simulink model "EvilSpagetty"  (R2020b)
settings: Solver=VariableStepAuto  StartTime=0.0  StopTime=3  RelTol=1e-3
(part 5 of 7)

== matlab function EvilSpagetty/1//Mt ==
  data: u1 input; y output; u2 input; u3 input; u4 input; u5 input; u6 input; u7 input; u8 input; u9 input; u10 input
function y = fcn(u1,u2,u3,u4,u5,u6,u7,u8,u9,u10)
theta1=u6;
theta2=u7;
theta3=u8;
theta4=u9;
theta5=u10;
M=[(4725330594848641*cos(2*theta2))/288230376151711744 - (1393797*cos(2*theta3))/22300745198530623141535718272648361505980416 - (12544169*cos(2*theta4))/22300745198530623141535718272648361505980416 - (3240011242931075*cos(2*theta5))/73786976294838206464 + (3825825015716409*sin(2*theta2))/147573952589676412928 + (2282168433090971*sin(2*theta5))/37778931862957161709568 + (3257081095467945*cos(theta3))/288230376151711744 + (7220698343344529*cos(theta4))/2305843009213693952 - (7028085605816175*sin(theta3))/590295810358705651712 + (5387337053181017*cos(theta3)*cos(theta4))/1152921504606846976 + (5571380563941847*cos(theta5)*sin(theta4))/9223372036854775808 - (5387337053181017*sin(theta3)*sin(theta4))/1152921504606846976 - (7988070105025833*sin(theta4)*sin(theta5))/4722366482869645213696 + (3257081095467945*cos(2*theta2)*cos(theta3))/288230376151711744 - (13937967*cos(2*theta2)*cos(theta4))/2787593149816327892691964784081045188247552 - (13937967*cos(2*theta3)*cos(theta4))/2787593149816327892691964784081045188247552 - (7028085605816175*cos(2*theta2)*sin(theta3))/590295810358705651712 - (7028085605816175*sin(2*theta2)*cos(theta3))/590295810358705651712 + (2787593*sin(2*theta2)*cos(theta5))/5575186299632655785383929568162090376495104 + (2787593*sin(2*theta3)*cos(theta5))/5575186299632655785383929568162090376495104 + (2787593*sin(2*theta4)*cos(theta5))/5575186299632655785383929568162090376495104 - (3257081095467945*sin(2*theta2)*sin(theta3))/288230376151711744 + (13937965*sin(2*theta2)*sin(theta4))/2787593149816327892691964784081045188247552 - (2854495*sin(2*theta2)*sin(theta5))/5708990770823839524233143877797980545530986496 + (13937965*sin(2*theta3)*sin(theta4))/2787593149816327892691964784081045188247552 - (2854495*sin(2*theta3)*sin(theta5))/5708990770823839524233143877797980545530986496 - (2854495*sin(2*theta4)*sin(theta5))/5708990770823839524233143877797980545530986496 - (8356542075167085*cos(2*theta2)*cos(2*theta3))/2305843009213693952 - (11150375*cos(2*theta2)*cos(2*theta4))/178405961588244985132285746181186892047843328 - (1393797*cos(2*theta2)*cos(2*theta5))/22300745198530623141535718272648361505980416 - (11150375*cos(2*theta3)*cos(2*theta4))/178405961588244985132285746181186892047843328 - (1393797*cos(2*theta3)*cos(2*theta5))/22300745198530623141535718272648361505980416 - (1393797*cos(2*theta4)*cos(2*theta5))/22300745198530623141535718272648361505980416 - (1007824040173657*cos(2*theta2)*sin(2*theta3))/288230376151711744 - (1007824040173657*cos(2*theta3)*sin(2*theta2))/288230376151711744 - (17126969*cos(2*theta2)*sin(2*theta5))/91343852333181432387730302044767688728495783936 - (cos(2*theta5)*sin(2*theta2))/91343852333181432387730302044767688728495783936 - (17126969*cos(2*theta3)*sin(2*theta5))/91343852333181432387730302044767688728495783936 - (cos(2*theta5)*sin(2*theta3))/91343852333181432387730302044767688728495783936 - (17126969*cos(2*theta4)*sin(2*theta5))/91343852333181432387730302044767688728495783936 - (cos(2*theta5)*sin(2*theta4))/91343852333181432387730302044767688728495783936 + (8356542075167085*sin(2*theta2)*sin(2*theta3))/2305843009213693952 + (11150373*sin(2*theta2)*sin(2*theta4))/178405961588244985132285746181186892047843328 + (11150373*sin(2*theta3)*sin(2*theta4))/178405961588244985132285746181186892047843328 + (1160499590055099*cos(2*theta2)*cos(2*theta3)*cos(2*theta4))/4611686018427387904 - (11150375*cos(2*theta2)*cos(2*theta3)*cos(2*theta5))/178405961588244985132285746181186892047843328 - (11150375*cos(2*theta2)*cos(2*theta4)*cos(2*theta5))/178405961588244985132285746181186892047843328 - (11150375*cos(2*theta3)*cos(2*theta4)*cos(2*theta5))/178405961588244985132285746181186892047843328 - (5959870363491779*cos(theta3)*sin(theta4)*sin(theta5))/2361183241434822606848 - (5959870363491779*cos(theta4)*sin(theta3)*sin(theta5))/2361183241434822606848 - (2695991646372651*cos(2*theta2)*cos(2*theta3)*sin(2*theta4))/9223372036854775808 - (2695991646372651*cos(2*theta2)*cos(2*theta4)*sin(2*theta3))/9223372036854775808 - (2695991646372651*cos(2*theta3)*cos(2*theta4)*sin(2*theta2))/9223372036854775808 - (5708989*cos(2*theta2)*cos(2*theta3)*sin(2*theta5))/91343852333181432387730302044767688728495783936 - (5708989*cos(2*theta2)*cos(2*theta4)*sin(2*theta5))/91343852333181432387730302044767688728495783936 - (5708989*cos(2*theta3)*cos(2*theta4)*sin(2*theta5))/91343852333181432387730302044767688728495783936 - (1160499590055099*cos(2*theta2)*sin(2*theta3)*sin(2*theta4))/4611686018427387904 - (1160499590055099*cos(2*theta3)*sin(2*theta2)*sin(2*theta4))/4611686018427387904 - (1160499590055099*cos(2*theta4)*sin(2*theta2)*sin(2*theta3))/4611686018427387904 + (11150373*cos(2*theta5)*sin(2*theta2)*sin(2*theta3))/178405961588244985132285746181186892047843328 + (11150373*cos(2*theta5)*sin(2*theta2)*sin(2*theta4))/178405961588244985132285746181186892047843328 + (11150373*cos(2*theta5)*sin(2*theta3)*sin(2*theta4))/178405961588244985132285746181186892047843328 + (2695991646372651*sin(2*theta2)*sin(2*theta3)*sin(2*theta4))/9223372036854775808 + (5708991*sin(2*theta2)*sin(2*theta3)*sin(2*theta5))/91343852333181432387730302044767688728495783936 + (5708991*sin(2*theta2)*sin(2*theta4)*sin(2*theta5))/91343852333181432387730302044767688728495783936 + (5708991*sin(2*theta3)*sin(2*theta4)*sin(2*theta5))/91343852333181432387730302044767688728495783936 + (5387337053181017*cos(2*theta2)*cos(theta3)*cos(theta4))/1152921504606846976 - (5387337053181017*cos(2*theta2)*sin(theta3)*sin(theta4))/1152921504606846976 - (5387337053181017*sin(2*theta2)*cos(theta3)*sin(theta4))/1152921504606846976 - (5387337053181017*sin(2*theta2)*cos(theta4)*sin(theta3))/1152921504606846976 + (3568119*cos(2*theta2)*sin(theta4)*sin(theta5))/1427247692705959881058285969449495136382746624 + (3568119*sin(2*theta2)*cos(theta4)*sin(theta5))/1427247692705959881058285969449495136382746624 + (3568119*cos(2*theta3)*sin(theta4)*sin(theta5))/1427247692705959881058285969449495136382746624 + (3568119*sin(2*theta3)*cos(theta4)*sin(theta5))/1427247692705959881058285969449495136382746624 + (7220698343344529*cos(2*theta2)*cos(2*theta3)*cos(theta4))/2305843009213693952 + (2787593*cos(2*theta2)*sin(2*theta3)*cos(theta5))/5575186299632655785383929568162090376495104 + (2787593*cos(2*theta3)*sin(2*theta2)*cos(theta5))/5575186299632655785383929568162090376495104 + (2787593*cos(2*theta2)*sin(2*theta4)*cos(theta5))/5575186299632655785383929568162090376495104 + (2787593*cos(2*theta4)*sin(2*theta2)*cos(theta5))/5575186299632655785383929568162090376495104 + (2787593*cos(2*theta3)*sin(2*theta4)*cos(theta5))/5575186299632655785383929568162090376495104 + (2787593*cos(2*theta4)*sin(2*theta3)*cos(theta5))/5575186299632655785383929568162090376495104 - (7220698343344529*cos(2*theta2)*sin(2*theta3)*sin(theta4))/2305843009213693952 - (7220698343344529*cos(2*theta3)*sin(2*theta2)*sin(theta4))/2305843009213693952 - (7220698343344529*sin(2*theta2)*sin(2*theta3)*cos(theta4))/2305843009213693952 + (8313573984755043*cos(theta3)*cos(theta5)*sin(theta4))/9223372036854775808 + (8313573984755043*cos(theta4)*cos(theta5)*sin(theta3))/9223372036854775808 - (4653258611581729*sin(2*theta2)*sin(2*theta3)*sin(2*theta4)*cos(theta5))/36893488147419103232 + (9004151162956663*sin(2*theta2)*sin(2*theta3)*sin(2*theta4)*sin(theta5))/18889465931478580854784 + (8313573984755043*cos(2*theta2)*cos(theta3)*cos(theta5)*sin(theta4))/9223372036854775808 + (8313573984755043*cos(2*theta2)*cos(theta4)*cos(theta5)*sin(theta3))/9223372036854775808 + (8313573984755043*sin(2*theta2)*cos(theta3)*cos(theta4)*cos(theta5))/9223372036854775808 - (3240011242931075*cos(2*theta2)*cos(2*theta3)*cos(2*theta4)*cos(2*theta5))/73786976294838206464 - (5959870363491779*cos(2*theta2)*cos(theta3)*sin(theta4)*sin(theta5))/2361183241434822606848 - (5959870363491779*cos(2*theta2)*cos(theta4)*sin(theta3)*sin(theta5))/2361183241434822606848 - (5959870363491779*sin(2*theta2)*cos(theta3)*cos(theta4)*sin(theta5))/2361183241434822606848 + (2282168433090971*cos(2*theta2)*cos(2*theta3)*cos(2*theta4)*sin(2*theta5))/37778931862957161709568 - (8313573984755043*sin(2*theta2)*cos(theta5)*sin(theta3)*sin(theta4))/9223372036854775808 + (3240011242931075*cos(2*theta2)*cos(2*theta5)*sin(2*theta3)*sin(2*theta4))/73786976294838206464 + (3240011242931075*cos(2*theta3)*cos(2*theta5)*sin(2*theta2)*sin(2*theta4))/73786976294838206464 + (3240011242931075*cos(2*theta4)*cos(2*theta5)*sin(2*theta2)*sin(2*theta3))/73786976294838206464 + (5959870363491779*sin(2*theta2)*sin(theta3)*sin(theta4)*sin(theta5))/2361183241434822606848 - (2282168433090971*cos(2*theta2)*sin(2*theta3)*sin(2*theta4)*sin(2*theta5))/37778931862957161709568 - (2282168433090971*cos(2*theta3)*sin(2*theta2)*sin(2*theta4)*sin(2*theta5))/37778931862957161709568 - (2282168433090971*cos(2*theta4)*sin(2*theta2)*sin(2*theta3)*sin(2*theta5))/37778931862957161709568 + (5571380563941847*cos(2*theta2)*cos(2*theta3)*cos(theta5)*sin(theta4))/9223372036854775808 + (5571380563941847*cos(2*theta2)*sin(2*theta3)*cos(theta4)*cos(theta5))/9223372036854775808 + (5571380563941847*cos(2*theta3)*sin(2*theta2)*cos(theta4)*cos(theta5))/9223372036854775808 - (7988070105025833*cos(2*theta2)*cos(2*theta3)*sin(theta4)*sin(theta5))/4722366482869645213696 - (7988070105025833*cos(2*theta2)*sin(2*theta3)*cos(theta4)*sin(theta5))/4722366482869645213696 - (7988070105025833*cos(2*theta3)*sin(2*theta2)*cos(theta4)*sin(theta5))/4722366482869645213696 - (5571380563941847*sin(2*theta2)*sin(2*theta3)*cos(theta5)*sin(theta4))/9223372036854775808 + (7988070105025833*sin(2*theta2)*sin(2*theta3)*sin(theta4)*sin(theta5))/4722366482869645213696 + (4653258611581729*cos(2*theta2)*cos(2*theta3)*sin(2*theta4)*cos(theta5))/36893488147419103232 + (4653258611581729*cos(2*theta2)*cos(2*theta4)*sin(2*theta3)*cos(theta5))/36893488147419103232 + (4653258611581729*cos(2*theta3)*cos(2*theta4)*sin(2*theta2)*cos(theta5))/36893488147419103232 - (9004151162956663*cos(2*theta2)*cos(2*theta3)*sin(2*theta4)*sin(theta5))/18889465931478580854784 - (9004151162956663*cos(2*theta2)*cos(2*theta4)*sin(2*theta3)*sin(theta5))/18889465931478580854784 - (9004151162956663*cos(2*theta3)*cos(2*theta4)*sin(2*theta2)*sin(theta5))/18889465931478580854784 + 1286385292365897/36028797018963968, (4529589740700877256066888313638240905^(1/2)*cos(theta5 - theta2 + atan(5959870363491779/2128274940097291008)))/4722366482869645213696 - (8137087333510384493879446320585584785^(1/2)*cos(theta2 + theta3 + theta5 + atan(7988070105025833/2852546848738225664)))/9444732965739290427392 - (2751907161015558652484843253829882841^(1/2)*cos(theta2 + theta3 + theta4 + 2*theta5 - atan(1658885756380710400/2282168433090971)))/37778931862957161709568 + (5676236795239861057681171752444277073^(1/2)*cos(theta2 + theta3 + theta4 - theta5 - atan(9004151162956663/2382468409129845248)))/37778931862957161709568 + (284438032584458775502903691778485^(1/2)*cos(theta2 + theta3 + theta4 + atan(2263187056021513/16712750130780854)))/18446744073709551616 - (5676236795239861057681171752444277073^(1/2)*cos(theta2 + theta3 + theta4 + theta5 + atan(9004151162956663/2382468409129845248)))/37778931862957161709568 + (5*1142305347429842326012493489620072169^(1/2)*cos(theta2 + atan(5343930864547884032/6049849466133601)))/151115727451828646838272 - (4529589740700877256066888313638240905^(1/2)*cos(theta2 + theta5 + atan(5959870363491779/2128274940097291008)))/4722366482869645213696 - (2751907161015558652484843253829882841^(1/2)*cos(theta2 + theta3 + theta4 - 2*theta5 + atan(1658885756380710400/2282168433090971)))/37778931862957161709568 + (8137087333510384493879446320585584785^(1/2)*cos(theta2 + theta3 - theta5 - atan(7988070105025833/2852546848738225664)))/9444732965739290427392 + (1463392722678766663194006713130961^(1/2)*cos(theta2 + theta3 + atan(8937783066759625/37195547536369344)))/4611686018427387904, (5676236795239861057681171752444277073^(1/2)*cos(theta2 + theta3 + theta4 - theta5 - atan(9004151162956663/2382468409129845248)))/37778931862957161709568 - (2751907161015558652484843253829882841^(1/2)*cos(theta2 + theta3 + theta4 + 2*theta5 - atan(1658885756380710400/2282168433090971)))/37778931862957161709568 - (8137087333510384493879446320585584785^(1/2)*cos(theta2 + theta3 + theta5 + atan(7988070105025833/2852546848738225664)))/9444732965739290427392 + (284438032584458775502903691778485^(1/2)*cos(theta2 + theta3 + theta4 + atan(2263187056021513/16712750130780854)))/18446744073709551616 - (5676236795239861057681171752444277073^(1/2)*cos(theta2 + theta3 + theta4 + theta5 + atan(9004151162956663/2382468409129845248)))/37778931862957161709568 - (2751907161015558652484843253829882841^(1/2)*cos(theta2 + theta3 + theta4 - 2*theta5 + atan(1658885756380710400/2282168433090971)))/37778931862957161709568 + (8137087333510384493879446320585584785^(1/2)*cos(theta2 + theta3 - theta5 - atan(7988070105025833/2852546848738225664)))/9444732965739290427392 + (1463392722678766663194006713130961^(1/2)*cos(theta2 + theta3 + atan(8937783066759625/37195547536369344)))/4611686018427387904,                      (5676236795239861057681171752444277073^(1/2)*cos(theta2 + theta3 + theta4 - theta5 - atan(9004151162956663/2382468409129845248)))/37778931862957161709568 - (2751907161015558652484843253829882841^(1/2)*cos(theta2 + theta3 + theta4 + 2*theta5 - atan(1658885756380710400/2282168433090971)))/37778931862957161709568 + (284438032584458775502903691778485^(1/2)*cos(theta2 + theta3 + theta4 + atan(2263187056021513/16712750130780854)))/18446744073709551616 - (5676236795239861057681171752444277073^(1/2)*cos(theta2 + theta3 + theta4 + theta5 + atan(9004151162956663/2382468409129845248)))/37778931862957161709568 - (2751907161015558652484843253829882841^(1/2)*cos(theta2 + theta3 + theta4 - 2*theta5 + atan(1658885756380710400/2282168433090971)))/37778931862957161709568, (8313573984755043*cos(theta2)*cos(theta5))/9223372036854775808 - (5959870363491779*cos(theta2)*sin(theta5))/2361183241434822606848 - (5571380563941847*cos(theta5)*sin(theta2)*sin(theta3))/9223372036854775808 - (1951319518623669*sin(theta2)*sin(theta3)*sin(theta4))/9223372036854775808 + (7988070105025833*sin(theta2)*sin(theta3)*sin(theta5))/4722366482869645213696 + (5571380563941847*cos(theta2)*cos(theta3)*cos(theta5))/9223372036854775808 + (1951319518623669*cos(theta2)*cos(theta3)*sin(theta4))/9223372036854775808 + (1951319518623669*cos(theta2)*cos(theta4)*sin(theta3))/9223372036854775808 + (1951319518623669*cos(theta3)*cos(theta4)*sin(theta2))/9223372036854775808 - (7988070105025833*cos(theta2)*cos(theta3)*sin(theta5))/4722366482869645213696 + (4653258611581729*cos(theta2)*cos(theta3)*cos(theta4)*cos(theta5))/36893488147419103232 - (9004151162956663*cos(theta2)*cos(theta3)*cos(theta4)*sin(theta5))/18889465931478580854784 - (4653258611581729*cos(theta2)*cos(theta5)*sin(theta3)*sin(theta4))/36893488147419103232 - (4653258611581729*cos(theta3)*cos(theta5)*sin(theta2)*sin(theta4))/36893488147419103232 - (4653258611581729*cos(theta4)*cos(theta5)*sin(theta2)*sin(theta3))/36893488147419103232 + (9004151162956663*cos(theta2)*sin(theta3)*sin(theta4)*sin(theta5))/18889465931478580854784 + (9004151162956663*cos(theta3)*sin(theta2)*sin(theta4)*sin(theta5))/18889465931478580854784 + (9004151162956663*cos(theta4)*sin(theta2)*sin(theta3)*sin(theta5))/18889465931478580854784;
                                                                                                                                                                                                                                                                                                                                                                                                                                                                                                                                                                                                                                                                                                                                                                                                                                                                                                                                                                                                                                                                                                                                                                                                                                                                                                                                                                                                                                                                                                                                                                                                                                                                                                                                                                                                                                                                                                                                                                                                                                                                                                                                                                                                                                                                                                                                                                                                                                                                                                                                                                                                                                                                                                                                                                                                                                                                                                                                                                                                                                                                                                                                                                                                                                                                                                                                                                                                                                                                                                                                                                                                                                                                                                                                                                                                                                                                                                                                                                                                                                                                                                                                                                                                                                                                                                                                                                                                                                                                                                                                                                                                                                                                                                                                                                                                                                                                                                                                                                                                                                                                                                                                                                                                                                                                                                                                                                                                                                                                                                                                                                                                                                                                                                                                                                                                                                                                                                                                                                                                                                                                                                                                                                                                                                                                                                                                                                                                                                                                                                                                                                                                                                                                                                                                                                                                                                                                                                                                                                                                                                                                                                                                                                                                                                                                                                                                                                                                                                                                                                                                                                                                                                                                                                                                                                                                                                                                                                                                                                                                                                                                                                                                                                                                                                                                                                                                                                                                                                                                                                                                                                                                                                                                                                                                                                                                                                                                                                                                                   (4529589740700877256066888313638240905^(1/2)*cos(theta5 - theta2 + atan(5959870363491779/2128274940097291008)))/4722366482869645213696 - (8137087333510384493879446320585584785^(1/2)*cos(theta2 + theta3 + theta5 + atan(7988070105025833/2852546848738225664)))/9444732965739290427392 - (2751907161015558652484843253829882841^(1/2)*cos(theta2 + theta3 + theta4 + 2*theta5 - atan(1658885756380710400/2282168433090971)))/37778931862957161709568 + (5676236795239861057681171752444277073^(1/2)*cos(theta2 + theta3 + theta4 - theta5 - atan(9004151162956663/2382468409129845248)))/37778931862957161709568 + (284438032584458775502903691778485^(1/2)*cos(theta2 + theta3 + theta4 + atan(2263187056021513/16712750130780854)))/18446744073709551616 - (5676236795239861057681171752444277073^(1/2)*cos(theta2 + theta3 + theta4 + theta5 + atan(9004151162956663/2382468409129845248)))/37778931862957161709568 + (5*1142305347429842326012493489620072169^(1/2)*cos(theta2 + atan(5343930864547884032/6049849466133601)))/151115727451828646838272 - (4529589740700877256066888313638240905^(1/2)*cos(theta2 + theta5 + atan(5959870363491779/2128274940097291008)))/4722366482869645213696 - (2751907161015558652484843253829882841^(1/2)*cos(theta2 + theta3 + theta4 - 2*theta5 + atan(1658885756380710400/2282168433090971)))/37778931862957161709568 + (8137087333510384493879446320585584785^(1/2)*cos(theta2 + theta3 - theta5 - atan(7988070105025833/2852546848738225664)))/9444732965739290427392 + (1463392722678766663194006713130961^(1/2)*cos(theta2 + theta3 + atan(8937783066759625/37195547536369344)))/4611686018427387904,                                                                                                                                                                                                                                                                                                                                                                                                                                                                                                                                                                                                                                                                                                                             (3257081095467945*cos(theta3))/144115188075855872 - (2282168433090971*sin(2*theta5))/18889465931478580854784 + (7220698343344529*cos(theta4))/1152921504606846976 - (7028085605816175*sin(theta3))/295147905179352825856 + (5387337053181017*cos(theta3)*cos(theta4))/576460752303423488 + (5571380563941847*cos(theta5)*sin(theta4))/4611686018427387904 - (5387337053181017*sin(theta3)*sin(theta4))/576460752303423488 - (7988070105025833*sin(theta4)*sin(theta5))/2361183241434822606848 + (3240011242931075*cos(theta5)^2)/18446744073709551616 - (5959870363491779*cos(theta3)*sin(theta4)*sin(theta5))/1180591620717411303424 - (5959870363491779*cos(theta4)*sin(theta3)*sin(theta5))/1180591620717411303424 + (8313573984755043*cos(theta3)*cos(theta5)*sin(theta4))/4611686018427387904 + (8313573984755043*cos(theta4)*cos(theta5)*sin(theta3))/4611686018427387904 + 2255979720785003901/36893488147419103232,                                                                                                                                                                                                                                                                                                     (3257081095467945*cos(theta3))/288230376151711744 - (2282168433090971*sin(2*theta5))/18889465931478580854784 + (7220698343344529*cos(theta4))/1152921504606846976 - (7028085605816175*sin(theta3))/590295810358705651712 + (5387337053181017*cos(theta3)*cos(theta4))/1152921504606846976 + (5571380563941847*cos(theta5)*sin(theta4))/4611686018427387904 - (5387337053181017*sin(theta3)*sin(theta4))/1152921504606846976 - (7988070105025833*sin(theta4)*sin(theta5))/2361183241434822606848 + (3240011242931075*cos(theta5)^2)/18446744073709551616 - (5959870363491779*cos(theta3)*sin(theta4)*sin(theta5))/2361183241434822606848 - (5959870363491779*cos(theta4)*sin(theta3)*sin(theta5))/2361183241434822606848 + (8313573984755043*cos(theta3)*cos(theta5)*sin(theta4))/9223372036854775808 + (8313573984755043*cos(theta4)*cos(theta5)*sin(theta3))/9223372036854775808 + 1045038663065800189/36893488147419103232, (7220698343344529*cos(theta4))/2305843009213693952 - (2282168433090971*sin(2*theta5))/18889465931478580854784 + (5387337053181017*cos(theta3)*cos(theta4))/1152921504606846976 + (5571380563941847*cos(theta5)*sin(theta4))/9223372036854775808 - (5387337053181017*sin(theta3)*sin(theta4))/1152921504606846976 - (7988070105025833*sin(theta4)*sin(theta5))/4722366482869645213696 + (3240011242931075*cos(theta5)^2)/18446744073709551616 - (5959870363491779*cos(theta3)*sin(theta4)*sin(theta5))/2361183241434822606848 - (5959870363491779*cos(theta4)*sin(theta3)*sin(theta5))/2361183241434822606848 + (8313573984755043*cos(theta3)*cos(theta5)*sin(theta4))/9223372036854775808 + (8313573984755043*cos(theta4)*cos(theta5)*sin(theta3))/9223372036854775808 + 180934087776586173/36893488147419103232,                                                                                                                                                                                                                                                                                                                                                                                                                                                                                                                                                                                                                                                                                                                                                                                                                                                                                                                                                                  (9004151162956663*cos(theta5))/18889465931478580854784 + (4653258611581729*sin(theta5))/36893488147419103232 + (7988070105025833*cos(theta4)*cos(theta5))/4722366482869645213696 + (5571380563941847*cos(theta4)*sin(theta5))/9223372036854775808 - (5959870363491779*cos(theta5)*sin(theta3)*sin(theta4))/2361183241434822606848 - (8313573984755043*sin(theta3)*sin(theta4)*sin(theta5))/9223372036854775808 + (5959870363491779*cos(theta3)*cos(theta4)*cos(theta5))/2361183241434822606848 + (8313573984755043*cos(theta3)*cos(theta4)*sin(theta5))/9223372036854775808;
                                                                                                                                                                                                                                                                                                                                                                                                                                                                                                                                                                                                                                                                                                                                                                                                                                                                                                                                                                                                                                                                                                                                                                                                                                                                                                                                                                                                                                                                                                                                                                                                                                                                                                                                                                                                                                                                                                                                                                                                                                                                                                                                                                                                                                                                                                                                                                                                                                                                                                                                                                                                                                                                                                                                                                                                                                                                                                                                                                                                                                                                                                                                                                                                                                                                                                                                                                                                                                                                                                                                                                                                                                                                                                                                                                                                                                                                                                                                                                                                                                                                                                                                                                                                                                                                                                                                                                                                                                                                                                                                                                                                                                                                                                                                                                                                                                                                                                                                                                                                                                                                                                                                                                                                                                                                                                                                                                                                                                                                                                                                                                                                                                                                                                                                                                                                                                                                                                                                                                                                                                                                                                                                                                                                                                                                                                                                                                                                                                                                                                                                                                                                                                                                                                                                                                                                                                                                                                                                                                                                                                                                                                                                                                                                                                                                                                                                                                                                                                                                                                                                                                                                                                                                                                                                                                                                                                                                                                                                                                                                                                                                                                                                                                                                                                                                                                                                                                                                                                                                                                                                                                                                                                                                                                                                                                                                                                                                                                                                                                                                                                                                                                                                                                                                                                                                                                                                                                         (5676236795239861057681171752444277073^(1/2)*cos(theta2 + theta3 + theta4 - theta5 - atan(9004151162956663/2382468409129845248)))/37778931862957161709568 - (2751907161015558652484843253829882841^(1/2)*cos(theta2 + theta3 + theta4 + 2*theta5 - atan(1658885756380710400/2282168433090971)))/37778931862957161709568 - (8137087333510384493879446320585584785^(1/2)*cos(theta2 + theta3 + theta5 + atan(7988070105025833/2852546848738225664)))/9444732965739290427392 + (284438032584458775502903691778485^(1/2)*cos(theta2 + theta3 + theta4 + atan(2263187056021513/16712750130780854)))/18446744073709551616 - (5676236795239861057681171752444277073^(1/2)*cos(theta2 + theta3 + theta4 + theta5 + atan(9004151162956663/2382468409129845248)))/37778931862957161709568 - (2751907161015558652484843253829882841^(1/2)*cos(theta2 + theta3 + theta4 - 2*theta5 + atan(1658885756380710400/2282168433090971)))/37778931862957161709568 + (8137087333510384493879446320585584785^(1/2)*cos(theta2 + theta3 - theta5 - atan(7988070105025833/2852546848738225664)))/9444732965739290427392 + (1463392722678766663194006713130961^(1/2)*cos(theta2 + theta3 + atan(8937783066759625/37195547536369344)))/4611686018427387904,                                                                                                                                                                                                                                                                                                                                                                                                                                                                                                                                                                                                                                                                                                                           (3257081095467945*cos(theta3))/288230376151711744 - (2282168433090971*sin(2*theta5))/18889465931478580854784 + (7220698343344529*cos(theta4))/1152921504606846976 - (7028085605816175*sin(theta3))/590295810358705651712 + (5387337053181017*cos(theta3)*cos(theta4))/1152921504606846976 + (5571380563941847*cos(theta5)*sin(theta4))/4611686018427387904 - (5387337053181017*sin(theta3)*sin(theta4))/1152921504606846976 - (7988070105025833*sin(theta4)*sin(theta5))/2361183241434822606848 + (3240011242931075*cos(theta5)^2)/18446744073709551616 - (5959870363491779*cos(theta3)*sin(theta4)*sin(theta5))/2361183241434822606848 - (5959870363491779*cos(theta4)*sin(theta3)*sin(theta5))/2361183241434822606848 + (8313573984755043*cos(theta3)*cos(theta5)*sin(theta4))/9223372036854775808 + (8313573984755043*cos(theta4)*cos(theta5)*sin(theta3))/9223372036854775808 + 1045038663065800189/36893488147419103232,                                                                                                                                                                                                                                                                                                                                                                                                                                                                                                                                                                                                                                                                                                                                                                                                                                                                   (7220698343344529*cos(theta4))/1152921504606846976 + (5571380563941847*cos(theta5)*sin(theta4))/4611686018427387904 - (2282168433090971*cos(theta5)*sin(theta5))/9444732965739290427392 - (7988070105025833*sin(theta4)*sin(theta5))/2361183241434822606848 + (3240011242931075*cos(theta5)^2)/18446744073709551616 + 1045038663065800189/36893488147419103232,                                                                                                                                                                                                                                                                                                                                                                                                                                                    (7220698343344529*cos(theta4))/2305843009213693952 + (5571380563941847*cos(theta5)*sin(theta4))/9223372036854775808 - (2282168433090971*cos(theta5)*sin(theta5))/9444732965739290427392 - (7988070105025833*sin(theta4)*sin(theta5))/4722366482869645213696 + (3240011242931075*cos(theta5)^2)/18446744073709551616 + 180934087776586173/36893488147419103232,                                                                                                                                                                                                                                                                                                                                                                                                                                                                                                                                                                                                                                                                                                                                                                                                                                                                                                                                                                                                                                                                                                                                                                                                                                                                                            (9004151162956663*cos(theta5))/18889465931478580854784 + (4653258611581729*sin(theta5))/36893488147419103232 + (7988070105025833*cos(theta4)*cos(theta5))/4722366482869645213696 + (5571380563941847*cos(theta4)*sin(theta5))/9223372036854775808;
                                                                                                                                                                                                                                                                                                                                                                                                                                                                                                                                                                                                                                                                                                                                                                                                                                                                                                                                                                                                                                                                                                                                                                                                                                                                                                                                                                                                                                                                                                                                                                                                                                                                                                                                                                                                                                                                                                                                                                                                                                                                                                                                                                                                                                                                                                                                                                                                                                                                                                                                                                                                                                                                                                                                                                                                                                                                                                                                                                                                                                                                                                                                                                                                                                                                                                                                                                                                                                                                                                                                                                                                                                                                                                                                                                                                                                                                                                                                                                                                                                                                                                                                                                                                                                                                                                                                                                                                                                                                                                                                                                                                                                                                                                                                                                                                                                                                                                                                                                                                                                                                                                                                                                                                                                                                                                                                                                                                                                                                                                                                                                                                                                                                                                                                                                                                                                                                                                                                                                                                                                                                                                                                                                                                                                                                                                                                                                                                                                                                                                                                                                                                                                                                                                                                                                                                                                                                                                                                                                                                                                                                                                                                                                                                                                                                                                                                                                                                                                                                                                                                                                                                                                                                                                                                                                                                                                                                                                                                                                                                                                                                                                                                                                                                                                                                                                                                                                                                                                                                                                                                                                                                                                                                                                                                                                                                                                                                                                                                                                                                                                                                                                                                                                                                                                                                                                                                                                                                                                                                                                                                                                                                                                                                                                                                                                                                              (5676236795239861057681171752444277073^(1/2)*cos(theta2 + theta3 + theta4 - theta5 - atan(9004151162956663/2382468409129845248)))/37778931862957161709568 - (2751907161015558652484843253829882841^(1/2)*cos(theta2 + theta3 + theta4 + 2*theta5 - atan(1658885756380710400/2282168433090971)))/37778931862957161709568 + (284438032584458775502903691778485^(1/2)*cos(theta2 + theta3 + theta4 + atan(2263187056021513/16712750130780854)))/18446744073709551616 - (5676236795239861057681171752444277073^(1/2)*cos(theta2 + theta3 + theta4 + theta5 + atan(9004151162956663/2382468409129845248)))/37778931862957161709568 - (2751907161015558652484843253829882841^(1/2)*cos(theta2 + theta3 + theta4 - 2*theta5 + atan(1658885756380710400/2282168433090971)))/37778931862957161709568,                                                                                                                                                                                                                                                                                                                                                                                                                                                                                                                                                                                                                                                                                                                                                                                                                                       (7220698343344529*cos(theta4))/2305843009213693952 - (2282168433090971*sin(2*theta5))/18889465931478580854784 + (5387337053181017*cos(theta3)*cos(theta4))/1152921504606846976 + (5571380563941847*cos(theta5)*sin(theta4))/9223372036854775808 - (5387337053181017*sin(theta3)*sin(theta4))/1152921504606846976 - (7988070105025833*sin(theta4)*sin(theta5))/4722366482869645213696 + (3240011242931075*cos(theta5)^2)/18446744073709551616 - (5959870363491779*cos(theta3)*sin(theta4)*sin(theta5))/2361183241434822606848 - (5959870363491779*cos(theta4)*sin(theta3)*sin(theta5))/2361183241434822606848 + (8313573984755043*cos(theta3)*cos(theta5)*sin(theta4))/9223372036854775808 + (8313573984755043*cos(theta4)*cos(theta5)*sin(theta3))/9223372036854775808 + 180934087776586173/36893488147419103232,                                                                                                                                                                                                                                                                                                                                                                                                                                                                                                                                                                                                                                                                                                                                                                                                                                                                    (7220698343344529*cos(theta4))/2305843009213693952 + (5571380563941847*cos(theta5)*sin(theta4))/9223372036854775808 - (2282168433090971*cos(theta5)*sin(theta5))/9444732965739290427392 - (7988070105025833*sin(theta4)*sin(theta5))/4722366482869645213696 + (3240011242931075*cos(theta5)^2)/18446744073709551616 + 180934087776586173/36893488147419103232,                                                                                                                                                                                                                                                                                                                                                                                                                                                                                                                                                                                                                                                       (3240011242931075*cos(theta5)^2)/18446744073709551616 - (2282168433090971*sin(2*theta5))/18889465931478580854784 + 180934087776586173/36893488147419103232,                                                                                                                                                                                                                                                                                                                                                                                                                                                                                                                                                                                                                                                                                                                                                                                                                                                                                                                                                                                                                                                                                                                                                                                                                                                                                                                                                                                                                                 (9004151162956663*cos(theta5))/18889465931478580854784 + (4653258611581729*sin(theta5))/36893488147419103232;
                                                                                                                                                                                                                                                                                                                                                                                                                                                                                                                                                                                                                                                                                                                                                                                                                                                                                                                                                                                                                                                                                                                                                                                                                                                                                                                                                                                                                                                                                                                                                                                                                                                                                                                                                                                                                                                                                                                                                                                                                                                                                                                                                                                                                                                                                                                                                                                                                                                                                                                                                                                                                                                                                                                                                                                                                                                                                                                                                                                                                                                                                                                                                                                                                                                                                                                                                                                                                                                                                                                                                                                                                                                                                                                                                                                                                                                                                                                                                                                                                                                                                                                                                                                                                                                                                                                                                                                                                                                                                                                                                                                                                                                                                                                                                                                                                                                                                                                                                                                                                                                                                                                                                                                                                                                                                                                                                                                                                                                                                                                                                                                                                                                                                                                                                                                                                                                                                                                                                                                                                                                                                                                                                                                                                                                                                                                                                                                                                                                                                                                                                                                                                                                                                                                                                                                                                                                                                                                                                                                                                                                                                                                                                                                                                                                                                                                                                                                                                                                                                                                                                                                                                                                                                                                                                                                                                                                                                                                                                                                                                                                                                                                                                                                                                                                                                                                                                                                                                                                                                                                                                                                                                                                                                                                                                                                                                                                                                                                                                                                                                                                                                                                                                                                                                                                                                                                                                                                                                                                                                                                                                                                                                                                                                                                                                                                                              (8313573984755043*cos(theta2)*cos(theta5))/9223372036854775808 - (5959870363491779*cos(theta2)*sin(theta5))/2361183241434822606848 - (5571380563941847*cos(theta5)*sin(theta2)*sin(theta3))/9223372036854775808 - (1951319518623669*sin(theta2)*sin(theta3)*sin(theta4))/9223372036854775808 + (7988070105025833*sin(theta2)*sin(theta3)*sin(theta5))/4722366482869645213696 + (5571380563941847*cos(theta2)*cos(theta3)*cos(theta5))/9223372036854775808 + (1951319518623669*cos(theta2)*cos(theta3)*sin(theta4))/9223372036854775808 + (1951319518623669*cos(theta2)*cos(theta4)*sin(theta3))/9223372036854775808 + (1951319518623669*cos(theta3)*cos(theta4)*sin(theta2))/9223372036854775808 - (7988070105025833*cos(theta2)*cos(theta3)*sin(theta5))/4722366482869645213696 + (4653258611581729*cos(theta2)*cos(theta3)*cos(theta4)*cos(theta5))/36893488147419103232 - (9004151162956663*cos(theta2)*cos(theta3)*cos(theta4)*sin(theta5))/18889465931478580854784 - (4653258611581729*cos(theta2)*cos(theta5)*sin(theta3)*sin(theta4))/36893488147419103232 - (4653258611581729*cos(theta3)*cos(theta5)*sin(theta2)*sin(theta4))/36893488147419103232 - (4653258611581729*cos(theta4)*cos(theta5)*sin(theta2)*sin(theta3))/36893488147419103232 + (9004151162956663*cos(theta2)*sin(theta3)*sin(theta4)*sin(theta5))/18889465931478580854784 + (9004151162956663*cos(theta3)*sin(theta2)*sin(theta4)*sin(theta5))/18889465931478580854784 + (9004151162956663*cos(theta4)*sin(theta2)*sin(theta3)*sin(theta5))/18889465931478580854784,                                                                                                                                                                                                                                                                                                                                                                                                                                                                                                                                                                                                                                                                                                                                                                                                                                                                                                                                                                                                                                                                            (9004151162956663*cos(theta5))/18889465931478580854784 + (4653258611581729*sin(theta5))/36893488147419103232 + (7988070105025833*cos(theta4)*cos(theta5))/4722366482869645213696 + (5571380563941847*cos(theta4)*sin(theta5))/9223372036854775808 - (5959870363491779*cos(theta5)*sin(theta3)*sin(theta4))/2361183241434822606848 - (8313573984755043*sin(theta3)*sin(theta4)*sin(theta5))/9223372036854775808 + (5959870363491779*cos(theta3)*cos(theta4)*cos(theta5))/2361183241434822606848 + (8313573984755043*cos(theta3)*cos(theta4)*sin(theta5))/9223372036854775808,                                                                                                                                                                                                                                                                                                                                                                                                                                                                                                                                                                                                                                                                                                                                                                                                                                                                                                                                                                                (9004151162956663*cos(theta5))/18889465931478580854784 + (4653258611581729*sin(theta5))/36893488147419103232 + (7988070105025833*cos(theta4)*cos(theta5))/4722366482869645213696 + (5571380563941847*cos(theta4)*sin(theta5))/9223372036854775808,                                                                                                                                                                                                                                                                                                                                                                                                                                                                                                                                                                                                                                                                                                     (9004151162956663*cos(theta5))/18889465931478580854784 + (4653258611581729*sin(theta5))/36893488147419103232,                                                                                                                                                                                                                                                                                                                                                                                                                                                                                                                                                                                                                                                                                                                                                                                                                                                                                                                                                                                                                                                                                                                                                                                                                                                                                                                                                                                                                                                                                                         1951319518623669/9223372036854775808];
Ms=inv(M);                                                                                                                                                                                                                                                                                                                                                                                                                                                                                                                                                                                                                                                                                                                                                                                                                                                                                                                                                                                                                                                                                                                                                                                                                                                                                                                                                                                                                                                                                                                                                                                                                                                                                                                                                                                                                                                                                                                                                                                                                                                                                                                                                                                                                                                                                                                                                                                                                                                                                                                                                                                                                                                                                                                                                                                                                                                                                                                                                                                                                                                                                                                                                                                                                                                                                                                                                                                                                                                                                                                                                                                                                                                                                                                                                                                                                                                                                                                                                                                                                                                                                                                                                                                                                                                                                                                                                                                                                                                                                                                                                                                                                                                                                                                                                                                                                                                                                                                                                                                                                                                                                                                                                                                                                                                                                                                                                                                                                                                                                                                                                                                                                                                                                                                                                                                                                                                                                                                                                                                                                                                                                                                                                                                                                                                                                                                                                                                                                                                                                                                                                                                                                                                                                                                                                                                                                                                                                                                                                                                                                                                                                                                                                                                                                                                                                                                                                                                                                                                                                                                                                                                                                                                                                                                                                                                                                                                                                                                                                                                                                                                                                                                                                                                                                                                                                                                                                                                                                                                                                                                                                                                                                                                                                                                                                                                                                                                                                                                                                                                                                                                                                                                                                                                                                                                                                                                                                                                                                                                                                                                                                                                                                                                                                                                                                                                                          
in=[u1;u2;u3;u4;u5];
Z=Ms*in;
y = Z
